simulink subsystem "completeSubSystem"  (R2020a)
settings: Solver=VariableStepAuto  StartTime=0.0  StopTime=10.0  RelTol=1e-3
libraries: simulink x2
settings Model: Creator=shrad  LastModifiedBy=shrad

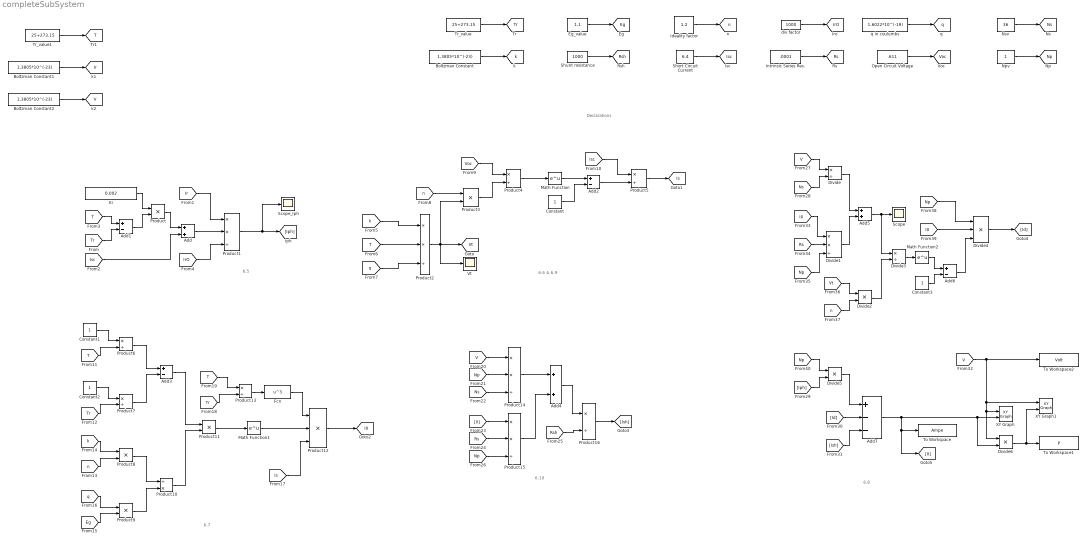
== system completeSubSystem ==
  note: 6.8
  note: 6.10
  note: 6.7
  note: 6.6 & 6.9
  note: 6.5
  note: Declarations
  Add : Sum
  Add{1..3,6} (4 alike) : Sum  Inputs=+-
  Add4 : Sum
  Add5 : Sum
  Add7 : Sum  Inputs=+--
  Boltzman Constant : Constant  Value=1.3805*10^(-23)
  Boltzman Constant1 : Constant  Value=1.3805*10^(-23)
  Boltzman Constant2 : Constant  Value=1.3805*10^(-23)
  Constant{,1..3} (4 alike) : Constant
  Divide : Product  Inputs=*/
  Divide1 : Product  Inputs=**/
  Divide2 : Product
  Divide3 : Product  Inputs=*/
  Divide4 : Product  Inputs=3
  Divide5 : Product
  Divide6 : Product
  Eg_value : Constant  Value=1.1
  Fcn : Fcn  Expr=u^3
  Ideality factor : Constant  Value=1.2
  Intrinsic Series Res. : Constant  Value=.0001
  Ki : Constant  Value=0.002
  Math Function : Math  SaturateOnIntegerOverflow=on
  Math Function1 : Math  SaturateOnIntegerOverflow=on
  Math Function2 : Math  SaturateOnIntegerOverflow=on
  Npv : Constant
  Nsv : Constant  Value=36
  Open Circuit Voltage : Constant  Value=.611
  Product : Product
  Product{1..2,14..15} (4 alike) : Product  Inputs=**/
  Product10 : Product  Inputs=/*
  Product11 : Product  Inputs=**
  Product12 : Product  Inputs=***
  Product{4..7,13,16} (6 alike) : Product  Inputs=*/
  Product3 : Product
  Product8 : Product  Inputs=**
  Product9 : Product  Inputs=**
  Scope : Scope
  Scope_Iph : Scope
  Short Circuit Current : Constant  Value=6.4
  Shunt resistance : Constant  Value=1000
  To Workspace : ToWorkspace  VariableName=Ampe  SaveFormat=Timeseries  SampleTime=-1
  To Workspace1 : ToWorkspace  VariableName=P  SaveFormat=Timeseries  SampleTime=-1
  To Workspace2 : ToWorkspace  VariableName=Volt  SaveFormat=Timeseries  SampleTime=-1
  Tr_value : Constant  Value=25+273.15
  Tr_value1 : Constant  Value=25+273.15
  Vt : Scope
  XY Graph : simulink/Sinks/XY Graph  xmin=-1  xmax=1  ymin=-1  ymax=1  st=-1
  XY Graph1 : simulink/Sinks/XY Graph  xmin=-1  xmax=1  ymin=-1  ymax=1  st=-1
  div factor : Constant  Value=1000
  q in coulumbs : Constant  Value=1.6022*10^(-19)
  tag scope: Eg=global, I0=global, Ir=global, IrO=global, Is=global, Isc=global, Np=global, Ns=global, Rs=global, Rsh=global, T=global, Tr=global, V=global, Voc=global, Vt=global, k=global, n=global, q=global
  wires:
  Short Circuit Current/1 -> [Isc]
  Shunt resistance/1 -> [Rsh]
  Tr_value/1 -> [Tr]
  Ideality factor/1 -> [n]
  div factor/1 -> [IrO]
  Eg_value/1 -> [Eg]
  Boltzman Constant/1 -> [k]
  Open Circuit Voltage/1 -> [Voc]
  q in coulumbs/1 -> [q]
  Add/1 -> Product1/2
  [Tr] -> Add1/2
  [IrO] -> Product1/3
  Ki/1 -> Product/1
  [Ir] -> Product1/1
  Product/1 -> Add/1
  Add1/1 -> Product/2
  Product1/1 -> Scope_Iph/1, [Iph]
  [Isc] -> Add/2
  [T] -> Add1/1
  Product4/1 -> Math Function/1
  Product2/1 -> Product3/2, Vt/1, [Vt]
  [k] -> Product2/1
  Math Function/1 -> Add2/1
  Add2/1 -> Product5/2
  [Voc] -> Product4/1
  [n] -> Product3/1
  Product5/1 -> [Is]
  [q] -> Product2/3
  [T] -> Product2/2
  [Isc] -> Product5/1
  Constant/1 -> Add2/2
  Product3/1 -> Product4/2
  Fcn/1 -> Product12/1
  [T] -> Product13/1
  Product12/1 -> [I0]
  Product9/1 -> Product10/2
  Constant2/1 -> Product7/1
  [Is] -> Product12/3
  [Tr] -> Product13/2
  Product11/1 -> Math Function1/1
  Math Function1/1 -> Product12/2
  Product10/1 -> Product11/2
  Add3/1 -> Product11/1
  Product7/1 -> Add3/2
  Product8/1 -> Product10/1
  [T] -> Product6/2
  [q] -> Product9/1
  Constant1/1 -> Product6/1
  [Eg] -> Product9/2
  Product13/1 -> Fcn/1
  [k] -> Product8/1
  [n] -> Product8/2
  [Tr] -> Product7/2
  Product6/1 -> Add3/1
  [Np] -> Product15/3
  [Rs] -> Product15/2
  [Rsh] -> Product16/2
  [II] -> Product15/1
  Product16/1 -> [Ish]
  [Ns] -> Product14/3
  Product14/1 -> Add4/1
  Add4/1 -> Product16/1
  [Np] -> Product14/2
  [V] -> Product14/1
  Product15/1 -> Add4/2
  Math Function2/1 -> Add6/1
  Add7/1 -> [II], To Workspace/1, Divide6/2, XY Graph/2
  Constant3/1 -> Add6/2
  [I0] -> Divide4/2
  Divide5/1 -> Add7/1
  [V] -> To Workspace2/1, XY Graph1/1, Divide6/1, XY Graph/1
  Divide2/1 -> Divide3/2
  Add5/1 -> Scope/1, Divide3/1
  [Id] -> Add7/2
  Divide3/1 -> Math Function2/1
  Divide6/1 -> To Workspace1/1, XY Graph1/2
  [V] -> Divide/1
  [Np] -> Divide5/1
  Add6/1 -> Divide4/3
  Divide1/1 -> Add5/2
  [I0] -> Divide1/1
  [Ns] -> Divide/2
  [Iph] -> Divide5/2
  [n] -> Divide2/2
  Divide/1 -> Add5/1
  [Ish] -> Add7/3
  [Np] -> Divide1/3
  Divide4/1 -> [Id]
  [Np] -> Divide4/1
  [Vt] -> Divide2/1
  [Rs] -> Divide1/2
  Npv/1 -> [Np]
  Nsv/1 -> [Ns]
  Intrinsic Series Res./1 -> [Rs]
  Boltzman Constant1/1 -> [Ir]
  Tr_value1/1 -> [T]
  Boltzman Constant2/1 -> [V]
